simulink model "BBB_USRLED_Test_LibraryBlock"  (R2013a)
settings: Solver=FixedStepDiscrete  StartTime=0.0  StopTime=inf  FixedStep=0.01  RelTol=1e-3
libraries: simulink x5, BLACKlink x4
settings Model: SimulationMode=external  ExtModeTrigDuration=100  Creator=rdustinkahawita  LastModifiedBy=rdustinkahawita
settings OptimizationCC: OptimizeModelRefInitCode=on  LifeSpan=1
settings DebuggingCC: SolverPrmCheckMsg=none  StrictBusMsg=Warning
settings HardwareCC: ProdLargestAtomicInteger=Long  ProdLargestAtomicFloat=Double  ProdEndianess=LittleEndian  ProdHWDeviceType=ARM Compatible->ARM Cortex
settings RTWCC: SystemTargetFile=realtime.tlc  GenerateMakefile=off  TemplateMakefile=realtime.tmf  Description=Run on Target Hardware  RTWVerbose=off  ProcessScript=realtime_make_rtw_hook
settings STFCustomTargetCC: TargetLibSuffix=.a  GenerateSampleERTMain=on  ERTCustomFileBanners=on  SupportNonInlinedSFcns=off  SupportVariableSizeSignals=on  MATLABClassNameForMDSCustomization=Simulink.SoftwareTarget.ERTCustomization  SystemTargetFile=realtime.tlc
settings ERTTargetCC: ParMdlRefBuildCompliant=off  CompOptLevelCompliant=off  ConcurrentExecutionCompliant=off  CombineOutputUpdateFcns=off  ERTFirstTimeCompliant=off  SupportContinuousTime=on  SupportVariableSizeSignals=on  ModelStepFunctionPrototypeControlCompliant=off  CPPClassGenCompliant=off  ExtMode=on  ExtModeMexArgs='192.168.7.2' 0 17725  ERTSrcFileBannerTemplate=realtime_code_template.cgt  ERTHdrFileBannerTemplate=realtime_code_template.cgt  ERTDataSrcFileTemplate=realtime_code_template.cgt  ERTDataHdrFileTemplate=realtime_code_template.cgt  ERTCustomFileTemplate=realtime_file_process.tlc

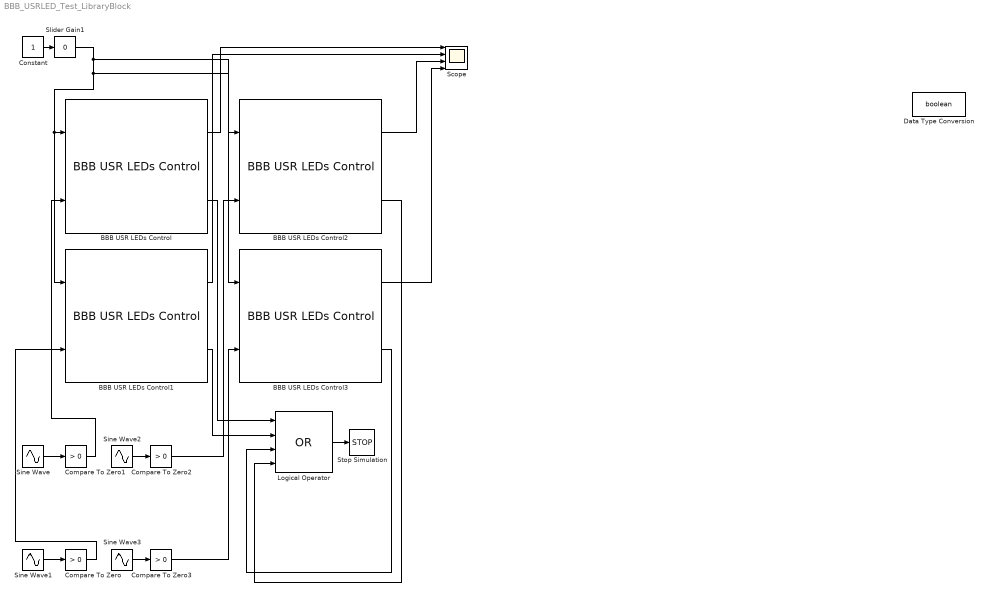
== system BBB_USRLED_Test_LibraryBlock ==
  BBB USR LEDs Control : BLACKlink/BBB USR LEDs Control  BBB_USRLED_No=USR0 LED  BBB_DebugInfo=Debug Level 2 - Include Diagnostics Info
  BBB USR LEDs Control1 : BLACKlink/BBB USR LEDs Control  BBB_USRLED_No=USR1 LED  BBB_DebugInfo=Debug Level 2 - Include Diagnostics Info
  BBB USR LEDs Control2 : BLACKlink/BBB USR LEDs Control  BBB_USRLED_No=USR2 LED  BBB_DebugInfo=Debug Level 2 - Include Diagnostics Info
  BBB USR LEDs Control3 : BLACKlink/BBB USR LEDs Control  BBB_USRLED_No=USR3 LED  BBB_DebugInfo=Debug Level 2 - Include Diagnostics Info
  Compare To Zero{,1..3} (4 alike) : simulink/Logic and Bit Operations/Compare To Zero  relop=>  OutDataTypeStr=boolean
  Constant : Constant
  Data Type Conversion : DataTypeConversion  OutDataTypeStr=boolean
  Logical Operator : Logic  Operator=OR  Inputs=4  AllPortsSameDT=off  OutDataTypeStr=boolean
  Scope : Scope  NumInputPorts=4
      settings: YMin=-5~-5~-5~-5  YMax=5~5~5~5
  Sine Wave : Sin  Frequency=5
  Sine Wave1 : Sin  Frequency=10
  Sine Wave2 : Sin  Frequency=15
  Sine Wave3 : Sin  Frequency=20
  Slider Gain1 : simulink/Math Operations/Slider Gain  low=0  gain=0  high=1
  Stop Simulation : Stop
  wires:
  BBB USR LEDs Control/2 -> Logical Operator/1
  BBB USR LEDs Control1/2 -> Logical Operator/2
  BBB USR LEDs Control3/2 -> Logical Operator/3
  BBB USR LEDs Control2/2 -> Logical Operator/4
  Logical Operator/1 -> Stop Simulation/1
  BBB USR LEDs Control/1 -> Scope/1
  BBB USR LEDs Control1/1 -> Scope/2
  BBB USR LEDs Control2/1 -> Scope/3
  BBB USR LEDs Control3/1 -> Scope/4
  Sine Wave1/1 -> Compare To Zero/1
  Compare To Zero/1 -> BBB USR LEDs Control1/2
  Sine Wave/1 -> Compare To Zero1/1
  Compare To Zero1/1 -> BBB USR LEDs Control/2
  Sine Wave2/1 -> Compare To Zero2/1
  Sine Wave3/1 -> Compare To Zero3/1
  Compare To Zero2/1 -> BBB USR LEDs Control2/2
  Compare To Zero3/1 -> BBB USR LEDs Control3/2
  Constant/1 -> Slider Gain1/1
  Slider Gain1/1 -> BBB USR LEDs Control1/1, BBB USR LEDs Control/1, BBB USR LEDs Control3/1, BBB USR LEDs Control2/1
